simulink model "Ejer8CalculoMinimos"  (R2023b)
settings: Solver=VariableStepAuto  StartTime=0.0  StopTime=10  RelTol=1e-3
undefined symbols (not defined in the file): my_fn
settings Model: Creator=alfre  LastModifiedBy=alfre

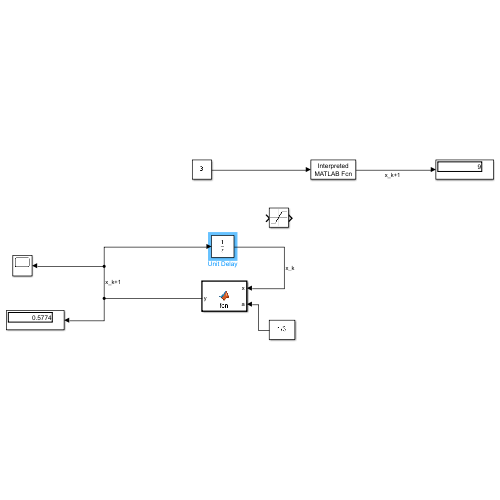
[thumbnail: Simulink's stored preview of the top-level diagram]
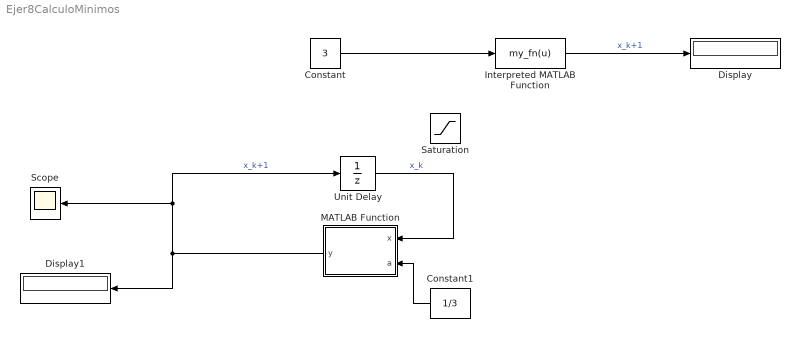
== system Ejer8CalculoMinimos ==
  Constant : Constant  Value=3
  Constant1 : Constant  Value=1/3
  Display : Display
  Display1 : Display
  Interpreted MATLAB Function : MATLABFcn  MATLABFcn=my_fn(u)
  MATLAB Function : MATLAB Function  TreatAsAtomicUnit=on
  Saturation : Saturate  UpperLimit=1  LowerLimit=0
  Scope : Scope
  Unit Delay : UnitDelay  SampleTime=-1  HasFrameUpgradeWarning=on
  wires:
  Interpreted MATLAB Function/1 -> Display/1  "x_k+1"
  Constant/1 -> Interpreted MATLAB Function/1
  MATLAB Function/1(y) -> Display1/1, Scope/1, Unit Delay/1  "x_k+1"
  Unit Delay/1 -> MATLAB Function/1(x)  "x_k"
  Constant1/1 -> MATLAB Function/2(a)

== matlab function Ejer8CalculoMinimos/MATLAB Function ==
  data: x input; y output; a input
function y = fcn(x, a)

y = x + a - x^2;
